simulink model "Different_K"  (R2021a)
settings: Solver=VariableStepAuto  StartTime=0.0  StopTime=10.0  RelTol=1e-3
libraries: fuzblock x6
settings Model: Creator=Anastasios  LastModifiedBy=Anastasios

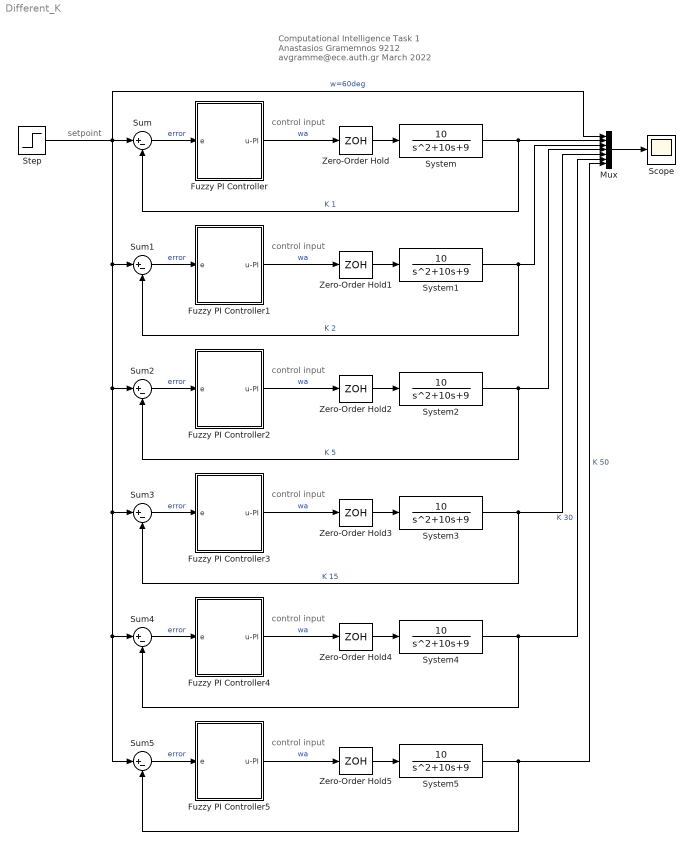
== system Different_K ==
  note: control input
  note: setpoint
  note: control input
  note: control input
  note: control input
  note: control input
  note: control input
  note: Computational Intelligence Task 1
      | Anastasios Gramemnos    9212
      | avgramme@ece.auth.gr    March 2022
  Fuzzy PI Controller : Subsystem
  Fuzzy PI Controller1 : Subsystem
  Fuzzy PI Controller2 : Subsystem
  Fuzzy PI Controller3 : Subsystem
  Fuzzy PI Controller4 : Subsystem
  Fuzzy PI Controller5 : Subsystem
  Mux : Mux  Inputs=7
  Scope : Scope
  Step : Step  Time=0  After=60  SampleTime=0.01
  Sum{,1..5} (6 alike) : Sum  Inputs=|+-
  System{,1..5} (6 alike) : TransferFcn  Numerator=[10]  Denominator=[1 10 9]
  Zero-Order Hold{,1..5} (6 alike) : ZeroOrderHold  SampleTime=0.01
  wires:
  Fuzzy PI Controller/1(u-PI) -> Zero-Order Hold/1  "wa"
  System/1 -> Sum/2, Mux/2  "K 1"
  Mux/1 -> Scope/1
  Zero-Order Hold/1 -> System/1
  Sum/1 -> Fuzzy PI Controller/1(e)  "error"
  Sum1/1 -> Fuzzy PI Controller1/1(e)  "error"
  Fuzzy PI Controller1/1(u-PI) -> Zero-Order Hold1/1  "wa"
  System1/1 -> Sum1/2, Mux/3  "K 2"
  Zero-Order Hold1/1 -> System1/1
  Sum2/1 -> Fuzzy PI Controller2/1(e)  "error"
  Fuzzy PI Controller2/1(u-PI) -> Zero-Order Hold2/1  "wa"
  System2/1 -> Sum2/2, Mux/4  "K 5"
  Zero-Order Hold2/1 -> System2/1
  Sum3/1 -> Fuzzy PI Controller3/1(e)  "error"
  Fuzzy PI Controller3/1(u-PI) -> Zero-Order Hold3/1  "wa"
  System3/1 -> Mux/5, Sum3/2  "K 15"
  Zero-Order Hold3/1 -> System3/1
  Sum4/1 -> Fuzzy PI Controller4/1(e)  "error"
  Fuzzy PI Controller4/1(u-PI) -> Zero-Order Hold4/1  "wa"
  System4/1 -> Mux/6, Sum4/2  "K 30"
  Zero-Order Hold4/1 -> System4/1
  Sum5/1 -> Fuzzy PI Controller5/1(e)  "error"
  Fuzzy PI Controller5/1(u-PI) -> Zero-Order Hold5/1  "wa"
  Step/1 -> Sum/1, Mux/1, Sum5/1, Sum4/1, Sum3/1, Sum2/1, Sum1/1  "w=60deg"
  System5/1 -> Mux/7, Sum5/2  "K 50"
  Zero-Order Hold5/1 -> System5/1

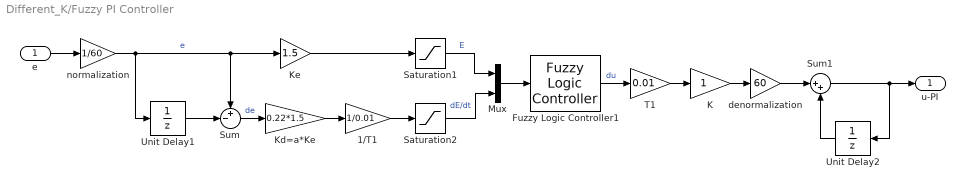
== system Different_K/Fuzzy PI Controller ==
  e : Inport
  1/T1 : Gain  Gain=1/0.01
  Fuzzy Logic Controller1 : fuzblock/Fuzzy Logic  Controller  FIS=FLC  OutputSampleNumber=101  DataType=double  FuzzifiedInputs=off  RuleFiringStrengths=off  RuleOutputs=off  AggregatedOutputs=off  SimulateUsing=Interpreted execution  OutOfRangeInputValueMessage=warning  NoRuleFiredMessage=warning  EmptyOutputFuzzySetMessage=warning
  K : Gain
  Kd=a*Ke : Gain  Gain=0.22*1.5
  Ke : Gain  Gain=1.5
  Mux : Mux  Inputs=2
  Saturation1 : Saturate  UpperLimit=1  LowerLimit=-1
  Saturation2 : Saturate  UpperLimit=1  LowerLimit=-1
  Sum : Sum  Inputs=+-|
  Sum1 : Sum  Inputs=|++
  T1 : Gain  Gain=0.01
  Unit Delay1 : UnitDelay  SampleTime=-1  HasFrameUpgradeWarning=on
  Unit Delay2 : UnitDelay  SampleTime=-1  HasFrameUpgradeWarning=on
  denormalization : Gain  Gain=60
  normalization : Gain  Gain=1/60
  u-PI : Outport
  wires:
  Unit Delay1/1 -> Sum/2
  normalization/1 -> Ke/1, Sum/1, Unit Delay1/1  "e"
  Sum/1 -> Kd=a*Ke/1  "de"
  Kd=a*Ke/1 -> 1/T1/1
  1/T1/1 -> Saturation2/1
  Ke/1 -> Saturation1/1
  Mux/1 -> Fuzzy Logic Controller1/1
  Saturation1/1 -> Mux/1  "E"
  Saturation2/1 -> Mux/2  "dE/dt"
  Fuzzy Logic Controller1/1 -> T1/1  "du"
  T1/1 -> K/1
  K/1 -> denormalization/1
  denormalization/1 -> Sum1/1
  Unit Delay2/1 -> Sum1/2
  Sum1/1 -> u-PI/1, Unit Delay2/1
  e/1 -> normalization/1

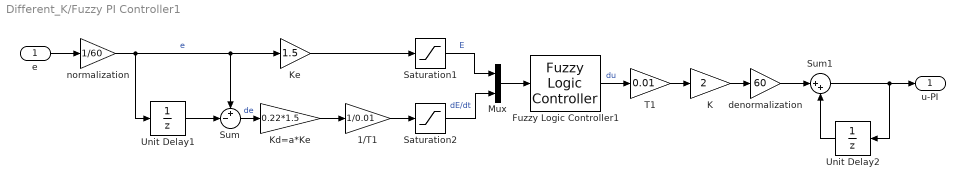
== system Different_K/Fuzzy PI Controller1 ==
  e : Inport
  1/T1 : Gain  Gain=1/0.01
  Fuzzy Logic Controller1 : fuzblock/Fuzzy Logic  Controller  FIS=FLC  OutputSampleNumber=101  DataType=double  FuzzifiedInputs=off  RuleFiringStrengths=off  RuleOutputs=off  AggregatedOutputs=off  SimulateUsing=Interpreted execution  OutOfRangeInputValueMessage=warning  NoRuleFiredMessage=warning  EmptyOutputFuzzySetMessage=warning
  K : Gain  Gain=2
  Kd=a*Ke : Gain  Gain=0.22*1.5
  Ke : Gain  Gain=1.5
  Mux : Mux  Inputs=2
  Saturation1 : Saturate  UpperLimit=1  LowerLimit=-1
  Saturation2 : Saturate  UpperLimit=1  LowerLimit=-1
  Sum : Sum  Inputs=+-|
  Sum1 : Sum  Inputs=|++
  T1 : Gain  Gain=0.01
  Unit Delay1 : UnitDelay  SampleTime=-1  HasFrameUpgradeWarning=on
  Unit Delay2 : UnitDelay  SampleTime=-1  HasFrameUpgradeWarning=on
  denormalization : Gain  Gain=60
  normalization : Gain  Gain=1/60
  u-PI : Outport
  wires:
  e/1 -> normalization/1
  Sum1/1 -> Unit Delay2/1, u-PI/1
  Unit Delay2/1 -> Sum1/2
  denormalization/1 -> Sum1/1
  K/1 -> denormalization/1
  T1/1 -> K/1
  Fuzzy Logic Controller1/1 -> T1/1  "du"
  Saturation2/1 -> Mux/2  "dE/dt"
  Saturation1/1 -> Mux/1  "E"
  Mux/1 -> Fuzzy Logic Controller1/1
  Ke/1 -> Saturation1/1
  1/T1/1 -> Saturation2/1
  Kd=a*Ke/1 -> 1/T1/1
  Sum/1 -> Kd=a*Ke/1  "de"
  normalization/1 -> Unit Delay1/1, Sum/1, Ke/1  "e"
  Unit Delay1/1 -> Sum/2

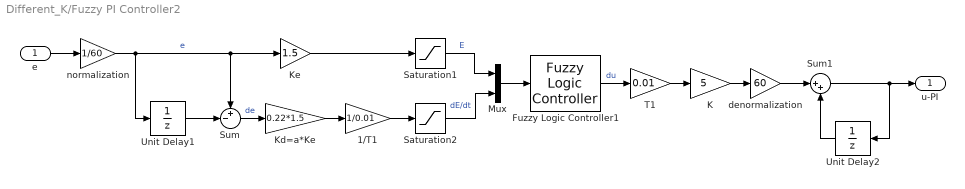
== system Different_K/Fuzzy PI Controller2 ==
  e : Inport
  1/T1 : Gain  Gain=1/0.01
  Fuzzy Logic Controller1 : fuzblock/Fuzzy Logic  Controller  FIS=FLC  OutputSampleNumber=101  DataType=double  FuzzifiedInputs=off  RuleFiringStrengths=off  RuleOutputs=off  AggregatedOutputs=off  SimulateUsing=Interpreted execution  OutOfRangeInputValueMessage=warning  NoRuleFiredMessage=warning  EmptyOutputFuzzySetMessage=warning
  K : Gain  Gain=5
  Kd=a*Ke : Gain  Gain=0.22*1.5
  Ke : Gain  Gain=1.5
  Mux : Mux  Inputs=2
  Saturation1 : Saturate  UpperLimit=1  LowerLimit=-1
  Saturation2 : Saturate  UpperLimit=1  LowerLimit=-1
  Sum : Sum  Inputs=+-|
  Sum1 : Sum  Inputs=|++
  T1 : Gain  Gain=0.01
  Unit Delay1 : UnitDelay  SampleTime=-1  HasFrameUpgradeWarning=on
  Unit Delay2 : UnitDelay  SampleTime=-1  HasFrameUpgradeWarning=on
  denormalization : Gain  Gain=60
  normalization : Gain  Gain=1/60
  u-PI : Outport
  wires:
  Unit Delay1/1 -> Sum/2
  normalization/1 -> Ke/1, Sum/1, Unit Delay1/1  "e"
  Sum/1 -> Kd=a*Ke/1  "de"
  Kd=a*Ke/1 -> 1/T1/1
  1/T1/1 -> Saturation2/1
  Ke/1 -> Saturation1/1
  Mux/1 -> Fuzzy Logic Controller1/1
  Saturation1/1 -> Mux/1  "E"
  Saturation2/1 -> Mux/2  "dE/dt"
  Fuzzy Logic Controller1/1 -> T1/1  "du"
  T1/1 -> K/1
  K/1 -> denormalization/1
  denormalization/1 -> Sum1/1
  Unit Delay2/1 -> Sum1/2
  Sum1/1 -> u-PI/1, Unit Delay2/1
  e/1 -> normalization/1

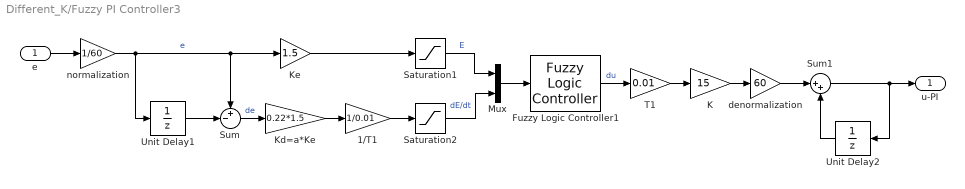
== system Different_K/Fuzzy PI Controller3 ==
  e : Inport
  1/T1 : Gain  Gain=1/0.01
  Fuzzy Logic Controller1 : fuzblock/Fuzzy Logic  Controller  FIS=FLC  OutputSampleNumber=101  DataType=double  FuzzifiedInputs=off  RuleFiringStrengths=off  RuleOutputs=off  AggregatedOutputs=off  SimulateUsing=Interpreted execution  OutOfRangeInputValueMessage=warning  NoRuleFiredMessage=warning  EmptyOutputFuzzySetMessage=warning
  K : Gain  Gain=15
  Kd=a*Ke : Gain  Gain=0.22*1.5
  Ke : Gain  Gain=1.5
  Mux : Mux  Inputs=2
  Saturation1 : Saturate  UpperLimit=1  LowerLimit=-1
  Saturation2 : Saturate  UpperLimit=1  LowerLimit=-1
  Sum : Sum  Inputs=+-|
  Sum1 : Sum  Inputs=|++
  T1 : Gain  Gain=0.01
  Unit Delay1 : UnitDelay  SampleTime=-1  HasFrameUpgradeWarning=on
  Unit Delay2 : UnitDelay  SampleTime=-1  HasFrameUpgradeWarning=on
  denormalization : Gain  Gain=60
  normalization : Gain  Gain=1/60
  u-PI : Outport
  wires:
  e/1 -> normalization/1
  Sum1/1 -> Unit Delay2/1, u-PI/1
  Unit Delay2/1 -> Sum1/2
  denormalization/1 -> Sum1/1
  K/1 -> denormalization/1
  T1/1 -> K/1
  Fuzzy Logic Controller1/1 -> T1/1  "du"
  Saturation2/1 -> Mux/2  "dE/dt"
  Saturation1/1 -> Mux/1  "E"
  Mux/1 -> Fuzzy Logic Controller1/1
  Ke/1 -> Saturation1/1
  1/T1/1 -> Saturation2/1
  Kd=a*Ke/1 -> 1/T1/1
  Sum/1 -> Kd=a*Ke/1  "de"
  normalization/1 -> Unit Delay1/1, Sum/1, Ke/1  "e"
  Unit Delay1/1 -> Sum/2

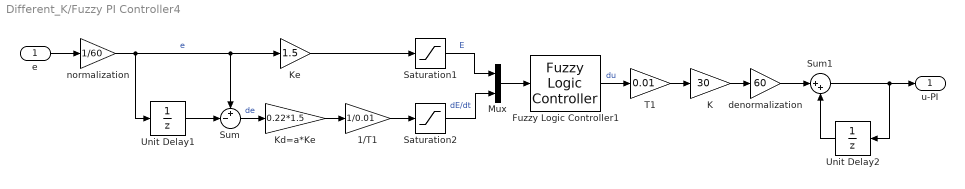
== system Different_K/Fuzzy PI Controller4 ==
  e : Inport
  1/T1 : Gain  Gain=1/0.01
  Fuzzy Logic Controller1 : fuzblock/Fuzzy Logic  Controller  FIS=FLC  OutputSampleNumber=101  DataType=double  FuzzifiedInputs=off  RuleFiringStrengths=off  RuleOutputs=off  AggregatedOutputs=off  SimulateUsing=Interpreted execution  OutOfRangeInputValueMessage=warning  NoRuleFiredMessage=warning  EmptyOutputFuzzySetMessage=warning
  K : Gain  Gain=30
  Kd=a*Ke : Gain  Gain=0.22*1.5
  Ke : Gain  Gain=1.5
  Mux : Mux  Inputs=2
  Saturation1 : Saturate  UpperLimit=1  LowerLimit=-1
  Saturation2 : Saturate  UpperLimit=1  LowerLimit=-1
  Sum : Sum  Inputs=+-|
  Sum1 : Sum  Inputs=|++
  T1 : Gain  Gain=0.01
  Unit Delay1 : UnitDelay  SampleTime=-1  HasFrameUpgradeWarning=on
  Unit Delay2 : UnitDelay  SampleTime=-1  HasFrameUpgradeWarning=on
  denormalization : Gain  Gain=60
  normalization : Gain  Gain=1/60
  u-PI : Outport
  wires:
  Unit Delay1/1 -> Sum/2
  normalization/1 -> Ke/1, Sum/1, Unit Delay1/1  "e"
  Sum/1 -> Kd=a*Ke/1  "de"
  Kd=a*Ke/1 -> 1/T1/1
  1/T1/1 -> Saturation2/1
  Ke/1 -> Saturation1/1
  Mux/1 -> Fuzzy Logic Controller1/1
  Saturation1/1 -> Mux/1  "E"
  Saturation2/1 -> Mux/2  "dE/dt"
  Fuzzy Logic Controller1/1 -> T1/1  "du"
  T1/1 -> K/1
  K/1 -> denormalization/1
  denormalization/1 -> Sum1/1
  Unit Delay2/1 -> Sum1/2
  Sum1/1 -> u-PI/1, Unit Delay2/1
  e/1 -> normalization/1

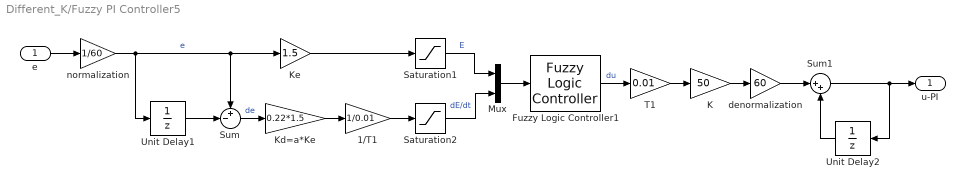
== system Different_K/Fuzzy PI Controller5 ==
  e : Inport
  1/T1 : Gain  Gain=1/0.01
  Fuzzy Logic Controller1 : fuzblock/Fuzzy Logic  Controller  FIS=FLC  OutputSampleNumber=101  DataType=double  FuzzifiedInputs=off  RuleFiringStrengths=off  RuleOutputs=off  AggregatedOutputs=off  SimulateUsing=Interpreted execution  OutOfRangeInputValueMessage=warning  NoRuleFiredMessage=warning  EmptyOutputFuzzySetMessage=warning
  K : Gain  Gain=50
  Kd=a*Ke : Gain  Gain=0.22*1.5
  Ke : Gain  Gain=1.5
  Mux : Mux  Inputs=2
  Saturation1 : Saturate  UpperLimit=1  LowerLimit=-1
  Saturation2 : Saturate  UpperLimit=1  LowerLimit=-1
  Sum : Sum  Inputs=+-|
  Sum1 : Sum  Inputs=|++
  T1 : Gain  Gain=0.01
  Unit Delay1 : UnitDelay  SampleTime=-1  HasFrameUpgradeWarning=on
  Unit Delay2 : UnitDelay  SampleTime=-1  HasFrameUpgradeWarning=on
  denormalization : Gain  Gain=60
  normalization : Gain  Gain=1/60
  u-PI : Outport
  wires:
  e/1 -> normalization/1
  Sum1/1 -> Unit Delay2/1, u-PI/1
  Unit Delay2/1 -> Sum1/2
  denormalization/1 -> Sum1/1
  K/1 -> denormalization/1
  T1/1 -> K/1
  Fuzzy Logic Controller1/1 -> T1/1  "du"
  Saturation2/1 -> Mux/2  "dE/dt"
  Saturation1/1 -> Mux/1  "E"
  Mux/1 -> Fuzzy Logic Controller1/1
  Ke/1 -> Saturation1/1
  1/T1/1 -> Saturation2/1
  Kd=a*Ke/1 -> 1/T1/1
  Sum/1 -> Kd=a*Ke/1  "de"
  normalization/1 -> Unit Delay1/1, Sum/1, Ke/1  "e"
  Unit Delay1/1 -> Sum/2
